simulink model "flightSDM_2016b"  (Simulink 8.8)
settings: Solver=VariableStepAuto  StartTime=0.0  StopTime=0.1  RelTol=1e-3
values from neighbouring files (symbols this model uses):
  alphaBP = [-0.174532925199 0 0.174532925199 0.349065850399 0.523598775598]    [aerodataSDM.mat]
  alphaBP_Cmq = [-0.0767944870878 -0.0543807851148 -0.0319670831418 -0.00955338116881 0.0128603208042 0.0352740227771 0.0576877247501 0.0801014267231 0.102515128696 0.124928830669 0.147342532642 0.169756234615 ... (20 elements, 1x20)]    [aerodataSDM.mat]
  CFx = [-0.059960266 -0.067440609 -0.048297904 -0.032440486 -0.010909865 -0.045147056 -0.056418925 -0.039318706 -0.033136767 -0.032505639 -0.055256253 -0.067898905 ... (105 elements, 5x3x7)]    [aerodataSDM.mat]
  CFz = [0.68128921 0.091383369 -0.526801776 -1.110916316 -1.591959578 0.589129449 0.005311526 -0.615162351 -1.219078441 -1.695308993 0.492304056 -0.08436359 ... (105 elements, 5x3x7)]    [aerodataSDM.mat]
  CMmShifted = [0.0271257549299 0.0901620686015 0.145783517203 0.19638659152 0.119100813365 -0.0753206258376 -0.00323126450923 0.05450470069 0.0857681696273 0.0253376541033 -0.182971831347 -0.100913984904 ... (105 elements, 5x3x7)]    [aerodataSDM.mat]
  CMq = [-1.68203724293 -2.01817028394 -2.10648295116 -2.0617711515 -2.02280764854 -1.9821056212 -1.6053442323 -1.46878486294 -1.81415098254 -2.33660774481 -2.43579197335 -1.68474558536 ... (200 elements, 20x10)]    [aerodataSDM.mat]
  dEBP = [-0.174532925199 0 0.174532925199]    [aerodataSDM.mat]
  machBP = [0.3 0.7 0.9 1 1.1 1.2 1.5]    [aerodataSDM.mat]
  machBP_Cmq = [0.2 0.305555555556 0.411111111111 0.516666666667 0.622222222222 0.727777777778 0.833333333333 0.938888888889 1.04444444444 1.15]    [aerodataSDM.mat]
  Ts = 0.01    [runner.m]
  x0 = [ U0 ; W0 ; Q0 ; Theta0 ; Z0 ; deTrim ; 0 ]    [runner.m]
undefined symbols (not defined in the file or in its folder): deTrim
libraries: simulink x1
settings Model: Creator=skysh  LastModifiedBy=skysh
settings DataIOCC: LimitDataPoints=off  SaveFormat=Dataset  SignalLoggingSaveFormat=Dataset  ReturnWorkspaceOutputs=on
settings OptimizationCC: LifeSpan=auto
settings DebuggingCC: UnderspecifiedInitializationDetection=Simplified  MergeDetectMultiDrivingBlocksExec=error  FcnCallInpInsideContextMsg=error  UnconnectedInputMsg=none  UnconnectedOutputMsg=none  UnconnectedLineMsg=none  StateNameClashWarn=none  SFUnexpectedBacktrackingDiag=error  SFNoUnconditionalDefaultTransitionDiag=error  SFExecutionAtInitializationDiag=warning
settings HardwareCC: ProdBitPerPointer=64  ProdBitPerSizeT=64  ProdBitPerPtrDiffT=64  ProdLargestAtomicFloat=Float  ProdIntDivRoundTo=Zero  ProdEndianess=LittleEndian  ProdWordSize=64  ProdHWDeviceType=Intel->x86-64 (Windows64)
settings ModelReferenceCC: EnableRefExpFcnMdlSchedulingChecks=off  PropagateSignalLabelsOutOfModel=on
settings SFSimCC: SimUseLocalCustomCode=on
settings RTWCC: RTWUseLocalCustomCode=on
settings GRTTargetCC: TargetLangStandard=C99 (ISO)  CombineOutputUpdateFcns=on  GRTInterface=off
settings ConfigComp: CovMetricSettings=dwe  CovSaveCumulativeToWorkspaceVar=off  CovSaveSingleToWorkspaceVar=off  CovExternalEMLEnable=on

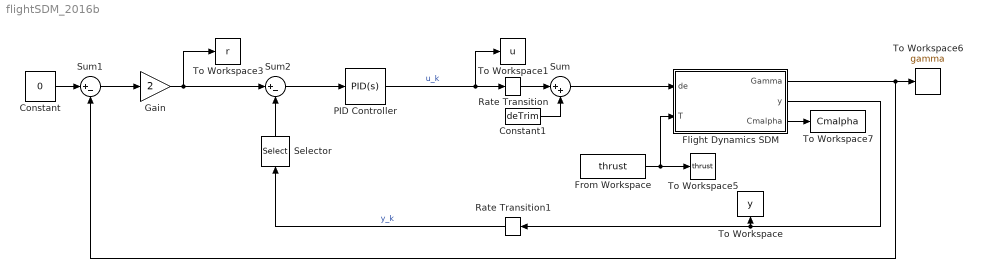
== system flightSDM_2016b ==
  Constant : Constant  Value=0
  Constant1 : Constant  Value=deTrim
  Flight Dynamics SDM : Subsystem
      mask Display: image('SDM.png');
  From Workspace : FromWorkspace  VariableName=thrust
  Gain : Gain  Gain=2
  PID Controller : simulink/Continuous/PID Controller  Controller=PID  Form=Parallel  TimeDomain=Continuous-time  SampleTime=-1  IntegratorMethod=Forward Euler  FilterMethod=Forward Euler  ControllerParametersSource=internal  P=-0.02  I=-2  D=0  N=100  UseFilter=on  InitialConditionSource=internal  InitialConditionForIntegrator=0  InitialConditionForFilter=0  DifferentiatorICPrevScaledInput=0  ExternalReset=none  TrackingMode=off  Kt=1  LimitOutput=on  UpperSaturationLimit=deg2rad(10)  LowerSaturationLimit=-deg2rad(10)  LinearizeAsGain=on  AntiWindupMode=none  Kb=1  POutMin=[]  POutMax=[]  IOutMin=[]  IOutMax=[]  DOutMin=[]  DOutMax=[]  NOutMin=[]  NOutMax=[]  SumOutMin=[]  SumOutMax=[]  SaturationOutMin=[]  SaturationOutMax=[]  PParamMin=[]  PParamMax=[]  IParamMin=[]  IParamMax=[]  DParamMin=[]  DParamMax=[]  NParamMin=[]  NParamMax=[]  KbParamMin=[]  KbParamMax=[]  KtParamMin=[]  KtParamMax=[]  KbOutMin=[]  KbOutMax=[]  KtOutMin=[]  KtOutMax=[]  IntegratorOutMin=[]  IntegratorOutMax=[]  FilterOutMin=[]  FilterOutMax=[]  SumI1OutMin=[]  SumI1OutMax=[]  SumI2OutMin=[]  SumI2OutMax=[]  SumI3OutMin=[]  SumI3OutMax=[]  SumDOutMin=[]  SumDOutMax=[]  DifferentiatorOutMin=[]  DifferentiatorOutMax=[]  IntegratorContinuousStateAttributes=''  IntegratorStateMustResolveToSignalObject=off  IntegratorRTWStateStorageClass=Auto  FilterContinuousStateAttributes=''  FilterStateMustResolveToSignalObject=off  FilterRTWStateStorageClass=Auto
  Rate Transition : RateTransition
  Rate Transition1 : RateTransition
  Selector : Selector  InputPortWidth=3  IndexOptions=Index vector (dialog)  Indices=[3]  OutputSizes=1
  Sum : Sum  Inputs=|++
  Sum1 : Sum  Inputs=|+-
  Sum2 : Sum  Inputs=|+-
  To Workspace : ToWorkspace  VariableName=y  SaveFormat=Structure With Time  SampleTime=Ts
  To Workspace1 : ToWorkspace  VariableName=u  SaveFormat=Structure With Time  SampleTime=Ts
  To Workspace3 : ToWorkspace  VariableName=r  SaveFormat=Structure With Time  SampleTime=Ts
  To Workspace5 : ToWorkspace  VariableName=thrust  SaveFormat=Structure With Time  SampleTime=Ts
  To Workspace6 : ToWorkspace  VariableName=gamma  SaveFormat=Structure With Time  SampleTime=Ts
  To Workspace7 : ToWorkspace  VariableName=Cmalpha  SaveFormat=Structure With Time  SampleTime=Ts
  wires:
  PID Controller/1 -> Rate Transition/1, To Workspace1/1  "u_k"
  Sum1/1 -> Gain/1
  Flight Dynamics SDM/2(y) -> To Workspace/1, Rate Transition1/1
  Constant1/1 -> Sum/2
  Sum/1 -> Flight Dynamics SDM/1(de)
  Rate Transition/1 -> Sum/1
  From Workspace/1 -> To Workspace5/1, Flight Dynamics SDM/2(T)
  Flight Dynamics SDM/1(Gamma) -> Sum1/2, To Workspace6/1
  Constant/1 -> Sum1/1
  Gain/1 -> Sum2/1, To Workspace3/1
  Flight Dynamics SDM/3(Cmalpha) -> To Workspace7/1
  Rate Transition1/1 -> Selector/1  "y_k"
  Selector/1 -> Sum2/2
  Sum2/1 -> PID Controller/1

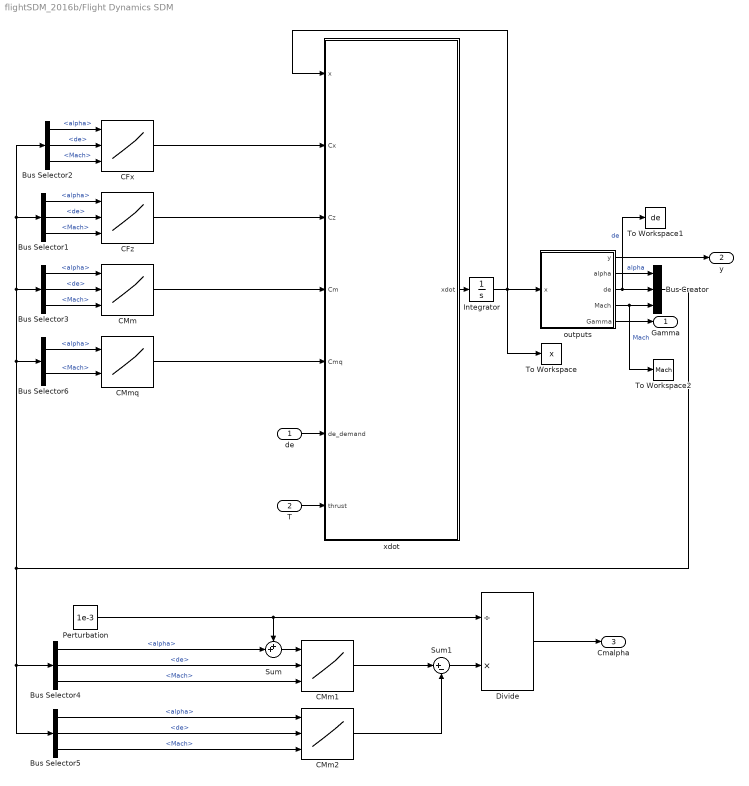
== system flightSDM_2016b/Flight Dynamics SDM ==
  de : Inport
  T : Inport  Port=2
  Bus Creator : BusCreator  Inputs=3
  Bus Selector{1..5} (5 alike) : BusSelector  OutputSignals=alpha,de,Mach
  Bus Selector6 : BusSelector  OutputSignals=alpha,Mach
  CFx : Lookup_n-D  NumberOfTableDimensions=3  BreakpointsForDimension1=alphaBP  BreakpointsForDimension2=dEBP  BreakpointsForDimension3=machBP  Table=CFx  InternalRulePriority=Speed  RndMeth=Simplest  InputSameDT=on
  CFz : Lookup_n-D  NumberOfTableDimensions=3  BreakpointsForDimension1=alphaBP  BreakpointsForDimension2=dEBP  BreakpointsForDimension3=machBP  Table=CFz  InternalRulePriority=Speed  RndMeth=Simplest  InputSameDT=on
  CMm : Lookup_n-D  NumberOfTableDimensions=3  BreakpointsForDimension1=alphaBP  BreakpointsForDimension2=dEBP  BreakpointsForDimension3=machBP  Table=CMmShifted  InternalRulePriority=Speed  RndMeth=Simplest  InputSameDT=on
  CMm1 : Lookup_n-D  NumberOfTableDimensions=3  BreakpointsForDimension1=alphaBP  BreakpointsForDimension2=dEBP  BreakpointsForDimension3=machBP  Table=CMmShifted  InternalRulePriority=Speed  RndMeth=Simplest  InputSameDT=on
  CMm2 : Lookup_n-D  NumberOfTableDimensions=3  BreakpointsForDimension1=alphaBP  BreakpointsForDimension2=dEBP  BreakpointsForDimension3=machBP  Table=CMmShifted  InternalRulePriority=Speed  RndMeth=Simplest  InputSameDT=on
  CMmq : Lookup_n-D  BreakpointsForDimension1=alphaBP_Cmq  BreakpointsForDimension2=machBP_Cmq  BreakpointsForDimension3=machBP  Table=CMq  InternalRulePriority=Speed  RndMeth=Simplest  InputSameDT=on
  Divide : Product  Inputs=/*
  Integrator : Integrator  InitialCondition=x0
  Perturbation : Constant  Value=1e-3
  Sum : Sum  Inputs=++|
  Sum1 : Sum  Inputs=|+-
  To Workspace : ToWorkspace  VariableName=x  SaveFormat=Structure With Time  SampleTime=Ts
  To Workspace1 : ToWorkspace  VariableName=de  SaveFormat=Structure With Time  SampleTime=Ts
  To Workspace2 : ToWorkspace  VariableName=Mach  SaveFormat=Structure With Time  SampleTime=Ts
  outputs : MATLAB Function  TreatAsAtomicUnit=on
  xdot : MATLAB Function  TreatAsAtomicUnit=on
  Gamma : Outport
  y : Outport  Port=2
  Cmalpha : Outport  Port=3
  wires:
  CFz/1 -> xdot/3(Cz)
  Bus Creator/1 -> Bus Selector6/1, Bus Selector3/1, Bus Selector1/1, Bus Selector2/1, Bus Selector5/1, Bus Selector4/1
  CFx/1 -> xdot/2(Cx)
  Bus Selector3/1 -> CMm/1  "<alpha>"
  CMm/1 -> xdot/4(Cm)
  outputs/2(alpha) -> Bus Creator/1  "alpha"
  xdot/1(xdot) -> Integrator/1
  Bus Selector3/2 -> CMm/2  "<de>"
  Bus Selector2/3 -> CFx/3  "<Mach>"
  Integrator/1 -> xdot/1(x), outputs/1(x), To Workspace/1
  Bus Selector2/1 -> CFx/1  "<alpha>"
  Bus Selector1/2 -> CFz/2  "<de>"
  outputs/1(y) -> y/1
  Bus Selector1/3 -> CFz/3  "<Mach>"
  Bus Selector1/1 -> CFz/1  "<alpha>"
  Bus Selector2/2 -> CFx/2  "<de>"
  outputs/3(de) -> Bus Creator/2, To Workspace1/1  "de"
  Bus Selector3/3 -> CMm/3  "<Mach>"
  outputs/4(Mach) -> To Workspace2/1, Bus Creator/3  "Mach"
  T/1 -> xdot/7(thrust)
  outputs/5(Gamma) -> Gamma/1
  Bus Selector4/2 -> CMm1/2  "<de>"
  Bus Selector4/3 -> CMm1/3  "<Mach>"
  Bus Selector5/1 -> CMm2/1  "<alpha>"
  Bus Selector5/2 -> CMm2/2  "<de>"
  Bus Selector5/3 -> CMm2/3  "<Mach>"
  Bus Selector4/1 -> Sum/2  "<alpha>"
  Sum/1 -> CMm1/1
  Perturbation/1 -> Sum/1, Divide/1
  CMm1/1 -> Sum1/1
  CMm2/1 -> Sum1/2
  Sum1/1 -> Divide/2
  Divide/1 -> Cmalpha/1
  de/1 -> xdot/6(de_demand)
  Bus Selector6/1 -> CMmq/1  "<alpha>"
  Bus Selector6/2 -> CMmq/2  "<Mach>"
  CMmq/1 -> xdot/5(Cmq)

== matlab function Flight Dynamics SDM/outputs ==
  data: x input double; y output double; alpha output double; de output double; Mach output double; Gamma output double
function [ y , alpha , de , Mach , Gamma ]= output(x)



coder.extrinsic('atmosisa');

U       = x(1);
W       = x(2); 
Theta   = x(4);
Z       = x(5); 
de      = x(6);

[~, a, ~, ~] = atmosisa(-Z);
Mach    = 0;
Mach    = sqrt(U^2 + W^2)/a;

alpha = atan2(W,U);
Gamma = Theta - alpha;

y = [ sqrt(U^2 + W^2 ) ; 
      alpha ;
      x(3) ];
% y = [ Speed;
%       alpha;
%       Q ]

== matlab function Flight Dynamics SDM/xdot ==
  data: x input double; Cx input double; xdot output double size=7; Cz input double; Cm input double; Cmq input double; de_demand input double; thrust input double; params parameter double
function xdot = flightdynamics(x,Cx,Cz,Cm,Cmq,de_demand,thrust,params)



coder.extrinsic('atmosisa');

m       = params.m;
g       = params.g; 
S       = params.S;
c       = params.c;
Jyy     = params.Jyy; 
Tx      = thrust;   


zeta_act  = params.zeta_act; 
omega_act = params.omega_act;   
udotlim   = params.udotlim;

 

U       = x(1);
W       = x(2);
Q       = x(3);
Theta   = x(4);
Z       = x(5); 

[~, ~ , ~, rho] = atmosisa(-Z);


q       = 0;
q       = 0.5*rho*( U^2 + W^2 );

alpha   = atan2(W,U);               %[rad]
sA      = sin(alpha);
cA      = cos(alpha);

sT = sin(Theta);
cT = cos(Theta);

[ CD , CL ] = rotate2wind( Cx , Cz , alpha );

D = q*S*CD;
L = q*S*CL;
M = q*S*c*Cm + q*S*c^2/2/( U^2 + W^2 )*Cmq;

xdot = zeros(7,1);

xdot(1) = ( -m*W*Q - cA*D + sA*L - m*g*sT + Tx )/m ; %U 
xdot(2) = (  m*U*Q - sA*D - cA*L + m*g*cT )/m; %W 
xdot(3) = ( M )/Jyy ; %Q 
xdot(4) = Q; %Theta
xdot(5) = -sin(Theta)*U + cos(Theta)*W; %Z


de_demand = min(deg2rad(10), max( de_demand, -deg2rad(10)));
x(6) = min(deg2rad(10), max( x(6), -deg2rad(10)));
x(7) = min(udotlim, max( x(7), -udotlim));
xdot(6) = x(7);
xdot(7) = -2*zeta_act*omega_act*x(7) - omega_act^2*x(6) + omega_act^2*de_demand;

end


function [ D  , L ] = rotate2wind( FX , FZ, alpha  )
Osa = [ cos(alpha)  sin(alpha);
       -sin(alpha)  cos(alpha)];
FW  = -1*Osa*[FX;FZ];
D = FW(1);
L = FW(2);
end
